simulink model "eVTOL_System"  (R2024b)
settings: Solver=FixedStepAuto  StartTime=0.0  StopTime=inf  RelTol=1e-3
undefined symbols (not defined in the file): airspeed, Battery, BCE12, BCE_Set_init, BMS_Controller_State, C, Cell10_P, Cell11_P, Cell12_P, Cell13_P, Cell14_P, Cell15_P, Cell16_P, Cell17_P, Cell18_P, Cell19_P, Cell1_N, Cell1_P, Cell20_P, Cell21_P, Cell22_P, Cell23_P, Cell24_P, Cell2_P, Cell3_P, Cell4_P, Cell5_P, Cell6_P, Cell7_P, Cell8_P, Cell9_P, Charging_State, CityMission, control, controlParams, ControlSampleTime, CriticalTiltAngle, currentFactor, CV_Gain, ddx, ddy, ddz, Device_01, Device_02, DiscIntNeverNeededParam, dx, dy, dz, Earth, env, F, F28379D_ADC_MaxCount, F28379D_ADC_Vmax, FixedWingMission, flightState, Foc_Ki_IxTcpu, Foc_Ki_S, Foc_Kp_I, Foc_Kp_S, fractalcoef ... (+68)
libraries: fl_lib x1115, nesl_utility x617, slrealtimeethercatlib x217, simulink x130, canmsglib x101, speedgoatlib_IO611_obsolete x91, slpidlib x49, mcbcontrolslib x44, slrealtimeutilitieslib x35, speedgoatlib_hdlCoder_IO3xx x31, dspstat3 x24, mcbpositiondecoderlib x12
(part 9 of 31)

== system eVTOL_System/Battery System/BMS/HIL/Controller_76Cells/Current Calculations ==
  BMS_Input : Inport
  Bus Selector : BusSelector  OutputSignals=Cell_Voltages,Cell_Temperatures
  Charge_Current_Limit_Calc : Subsystem
  Discharge_Current_Limit_Calc : Subsystem
  MinMax : MinMax
  MinMax1 : MinMax
  MinMax2 : MinMax  Function=max
  MinMax4 : MinMax  Function=max
  Selector1 : Subsystem
  Selector3 : Subsystem
  Discharge_Current_Limit : Outport
  Charge_Current_Limit : Outport  Port=2
  wires:
  MinMax/1 -> Discharge_Current_Limit_Calc/1(MinCellVolt)  "Min_Cell_Volt"
  MinMax4/1 -> Discharge_Current_Limit_Calc/3(MaxCellTemp), Charge_Current_Limit_Calc/3(MaxCellTemp)  "Max_Cell_Temp"
  MinMax1/1 -> Discharge_Current_Limit_Calc/2(MinCellTemp), Charge_Current_Limit_Calc/2(MinCellTemp)  "Min_Cell_Temp"
  MinMax2/1 -> Charge_Current_Limit_Calc/1(MaxCellVolt)  "Max_Cell_Volt"
  Discharge_Current_Limit_Calc/1(Discharge_Current_Limit) -> Discharge_Current_Limit/1  "Discharge_Current_Limit"
  Charge_Current_Limit_Calc/1(Charge_Current_Limit) -> Charge_Current_Limit/1  "Charge_Current_Limit"
  Bus Selector/1 -> Selector3/1(In1)  "<Cell_Voltages>"
  Bus Selector/2 -> Selector1/1(In1)  "<Cell_Temperatures>"
  BMS_Input/1 -> Bus Selector/1
  Selector3/1(Out1) -> MinMax/1, MinMax2/1
  Selector1/1(Out1) -> MinMax4/1, MinMax1/1

== system eVTOL_System/Battery System/BMS/HIL/Controller_76Cells/SOC Calculation ==
  BMS_State : Inport  OutDataTypeStr=Enum: BMS_Controller_State
  Sensor_Values : Inport  Port=2
  Bus Selector2 : BusSelector  OutputSignals=Pack_Current,Cell_Voltages,Cell_Temperatures
  Compare To Constant : simulink/Logic and Bit Operations/Compare To Constant  relop=~=  const=BMS_Controller_State.BMS_Fault  OutDataTypeStr=boolean
  Coulomb Counting : Subsystem  VariantControl=SocAlgo==1
  Gain : Gain  Gain=100
  Measurement Function : Subsystem  TreatAsAtomicUnit=on
  Mux : Mux  Inputs=3
  PackCurrent : Gain  Gain=-1
  Selector : Subsystem
  Selector1 : Subsystem
  State Transition Function : Subsystem  TreatAsAtomicUnit=on
  Temp : Selector  InputPortWidth=76  IndexOptions=Index vector (dialog)  Indices=1  OutputSizes=1
  UKF_EKF_1TC : Subsystem  VariantControl=CellType==1
  Volt : Selector  InputPortWidth=76  IndexOptions=Index vector (dialog)  Indices=1  OutputSizes=1
  SOC : Outport  OutDataTypeStr=single  VectorParamsAs1DForOutWhenUnconnected=off
  wires:
  Mux/1 -> Gain/1  "SOC"
  UKF_EKF_1TC/1(SOC_UKF) -> Mux/2  "SOC_UKF"
  BMS_State/1 -> Compare To Constant/1
  Coulomb Counting/1(SOC) -> Mux/1  "SOC_CC"
  Volt/1 -> UKF_EKF_1TC/1(Cell_Voltage)
  Temp/1 -> Coulomb Counting/2(Temp), State Transition Function/2(Temperature K), Measurement Function/2(Temperature (K))
  Compare To Constant/1 -> UKF_EKF_1TC/Enable
  UKF_EKF_1TC/2(SOC_EKF) -> Mux/3  "SOC_EKF"
  Bus Selector2/1 -> Coulomb Counting/1(Curr), PackCurrent/1  "<Pack_Current>"
  PackCurrent/1 -> State Transition Function/1(Current), Measurement Function/1(Current)  "PackCurrent"
  Bus Selector2/3 -> Selector1/1(In1)  "<Cell_Temperatures>"
  Bus Selector2/2 -> Selector/1(In1)  "<Cell_Voltages>"
  Sensor_Values/1 -> Bus Selector2/1
  Gain/1 -> SOC/1
  Selector/1(Out1) -> Volt/1
  Selector1/1(Out1) -> Temp/1

== system eVTOL_System/Battery System/BMS/MIL/Cell Monitoring Unit/Balancing_Circuit ==
  Bal_Cmd_Controller : Inport
  24-Cell : Subsystem  VariantControl=Ns_Module == 12
  Cells : PMIOPort  Side=Left
  Balancing_Currents : Outport
  wires:
  Bal_Cmd_Controller/1 -> 24-Cell/1(Bal_Cmd_Controller)
  24-Cell/1(Balancing_Currents) -> Balancing_Currents/1
  connections:
  Cells/RConn1 -- 24-Cell/LConn1

== system eVTOL_System/Battery System/BMS/MIL/Cell Monitoring Unit/Balancing_Circuit1 ==
  Bal_Cmd_Controller : Inport
  38-Cell : Subsystem  VariantControl=Ns_Module == 12
  Cells : PMIOPort  Side=Left
  Balancing_Currents : Outport
  wires:
  Bal_Cmd_Controller/1 -> 38-Cell/1(Bal_Cmd_Controller)
  38-Cell/1(Balancing_Currents) -> Balancing_Currents/1
  connections:
  Cells/RConn1 -- 38-Cell/LConn1

== system eVTOL_System/Battery System/BMS/MIL/Cell Monitoring Unit/Balancing_Circuit2 ==
  Bal_Cmd_Controller : Inport
  38-Cell : Subsystem  VariantControl=Ns_Module == 12
  Cells : PMIOPort  Side=Left
  Balancing_Currents : Outport
  wires:
  Bal_Cmd_Controller/1 -> 38-Cell/1(Bal_Cmd_Controller)
  38-Cell/1(Balancing_Currents) -> Balancing_Currents/1
  connections:
  Cells/RConn1 -- 38-Cell/LConn1

== system eVTOL_System/Battery System/BMS/MIL/Controller/BMS State Machine ==
  Discharge_Current_Limit : Inport
  Charge_Current_Limit : Inport  Port=2
  State_Request : Inport  Port=3  OutDataTypeStr=Enum: SRE
  Sensor_Values : Inport  Port=4
  Fault_Reset_Enable : Inport  Port=5
  Bus Selector : BusSelector  OutputSignals=Cell_Voltages,Pack_Voltage,Cell_Temperatures,Pack_Current
  Data Type Conversion : DataTypeConversion  OutDataTypeStr=boolean  SaturateOnIntegerOverflow=off  RndMeth=Floor
  State_Machine : Stateflow chart  TreatAsAtomicUnit=on  VariantControl=(default)
  Charge_Current_Req : Outport  OutMin=-100  OutMax=100  OutDataTypeStr=single  VectorParamsAs1DForOutWhenUnconnected=off
  Faults : Outport  Port=2  OutDataTypeStr=Bus: Faults  VectorParamsAs1DForOutWhenUnconnected=off  BusOutputAsStruct=on
  Charging_State : Outport  Port=3
  BMS_State : Outport  Port=4  OutDataTypeStr=Enum: BMS_Controller_State  VectorParamsAs1DForOutWhenUnconnected=off
  wires:
  State_Machine/2(Fault_out) -> Faults/1  "Faults"
  Bus Selector/1 -> State_Machine/4(Cell_Voltages)  "<Cell_Voltages>"
  State_Machine/1(ChargeCurrentReq) -> Charge_Current_Req/1  "Charge_Current_Req"
  State_Request/1 -> State_Machine/3(State_Request)
  Discharge_Current_Limit/1 -> State_Machine/1(DischargeCurrentLimit)
  Charge_Current_Limit/1 -> State_Machine/2(ChargeCurrentLimit)
  Bus Selector/3 -> State_Machine/6(Cell_Temperatures)  "<Cell_Temperatures>"
  Bus Selector/2 -> State_Machine/5(Pack_Voltage)  "<Pack_Voltage>"
  Bus Selector/4 -> State_Machine/7(Pack_Current)  "<Pack_Current>"
  Sensor_Values/1 -> Bus Selector/1
  Fault_Reset_Enable/1 -> Data Type Conversion/1
  Data Type Conversion/1 -> State_Machine/8(Fault_Reset_Enable)
  State_Machine/3(ChargeModeReq) -> Charging_State/1  "Charging_State"
  State_Machine/4(BMS_State) -> BMS_State/1  "BMS_State"

== system eVTOL_System/Battery System/BMS/MIL/Controller/Balancing Logic ==
  BMS_State : Inport  OutDataTypeStr=Enum: BMS_Controller_State  PortDimensions=1
  Sensor_Values : Inport  Port=2
  Balancing : Stateflow chart  TreatAsAtomicUnit=on  VariantControl=(default)
  Bus Selector1 : BusSelector  OutputSignals=Cell_Voltages
  Bal_Cmd : Outport  OutDataTypeStr=boolean  PortDimensions=[1,NumModules*Ns_Module]  VectorParamsAs1DForOutWhenUnconnected=off
  wires:
  Balancing/1(Bal_Cmd) -> Bal_Cmd/1  "Bal_Cmd"
  Bus Selector1/1 -> Balancing/2(CellVoltages)  "<Cell_Voltages>"
  Sensor_Values/1 -> Bus Selector1/1
  BMS_State/1 -> Balancing/1(BMS_State)

== system eVTOL_System/Battery System/BMS/MIL/Controller/Current Calculations ==
  BMS_Input : Inport
  Bus Selector : BusSelector  OutputSignals=Cell_Voltages,Cell_Temperatures
  Charge_Current_Limit_Calc : Subsystem
  Discharge_Current_Limit_Calc : Subsystem
  MinMax : MinMax
  MinMax1 : MinMax
  MinMax2 : MinMax  Function=max
  MinMax4 : MinMax  Function=max
  Discharge_Current_Limit : Outport
  Charge_Current_Limit : Outport  Port=2
  wires:
  MinMax/1 -> Discharge_Current_Limit_Calc/1(MinCellVolt)  "Min_Cell_Volt"
  MinMax4/1 -> Discharge_Current_Limit_Calc/3(MaxCellTemp), Charge_Current_Limit_Calc/3(MaxCellTemp)  "Max_Cell_Temp"
  MinMax1/1 -> Discharge_Current_Limit_Calc/2(MinCellTemp), Charge_Current_Limit_Calc/2(MinCellTemp)  "Min_Cell_Temp"
  MinMax2/1 -> Charge_Current_Limit_Calc/1(MaxCellVolt)  "Max_Cell_Volt"
  Discharge_Current_Limit_Calc/1(Discharge_Current_Limit) -> Discharge_Current_Limit/1  "Discharge_Current_Limit"
  Charge_Current_Limit_Calc/1(Charge_Current_Limit) -> Charge_Current_Limit/1  "Charge_Current_Limit"
  Bus Selector/1 -> MinMax/1, MinMax2/1  "<Cell_Voltages>"
  Bus Selector/2 -> MinMax4/1, MinMax1/1  "<Cell_Temperatures>"
  BMS_Input/1 -> Bus Selector/1

== system eVTOL_System/Battery System/BMS/MIL/Controller/SOC Calculation ==
  BMS_State : Inport  OutDataTypeStr=Enum: BMS_Controller_State
  Sensor_Values : Inport  Port=2
  Bus Selector2 : BusSelector  OutputSignals=Pack_Current,Cell_Voltages,Cell_Temperatures
  Compare To Constant : simulink/Logic and Bit Operations/Compare To Constant  relop=~=  const=BMS_Controller_State.BMS_Fault  OutDataTypeStr=boolean
  Coulomb Counting : Subsystem  VariantControl=SocAlgo==1
  Gain : Gain  Gain=100
  Measurement Function : Subsystem  TreatAsAtomicUnit=on
  Mux : Mux  Inputs=3
  PackCurrent : Gain  Gain=-1
  State Transition Function : Subsystem  TreatAsAtomicUnit=on
  Temp : Selector  InputPortWidth=Ns_Module*NumModules  IndexOptions=Index vector (dialog)  Indices=1  OutputSizes=1
  UKF_EKF_1TC : Subsystem  VariantControl=CellType==1
  Volt : Selector  InputPortWidth=Ns_Module*NumModules  IndexOptions=Index vector (dialog)  Indices=1  OutputSizes=1
  SOC : Outport  OutDataTypeStr=single  VectorParamsAs1DForOutWhenUnconnected=off
  wires:
  Mux/1 -> Gain/1  "SOC"
  UKF_EKF_1TC/1(SOC_UKF) -> Mux/2  "SOC_UKF"
  BMS_State/1 -> Compare To Constant/1
  Coulomb Counting/1(SOC) -> Mux/1  "SOC_CC"
  Volt/1 -> UKF_EKF_1TC/1(Cell_Voltage)
  Temp/1 -> Coulomb Counting/2(Temp), State Transition Function/2(Temperature K), Measurement Function/2(Temperature (K))
  Compare To Constant/1 -> UKF_EKF_1TC/Enable
  UKF_EKF_1TC/2(SOC_EKF) -> Mux/3  "SOC_EKF"
  Bus Selector2/1 -> Coulomb Counting/1(Curr), PackCurrent/1  "<Pack_Current>"
  PackCurrent/1 -> State Transition Function/1(Current), Measurement Function/1(Current)  "PackCurrent"
  Bus Selector2/3 -> Temp/1  "<Cell_Temperatures>"
  Bus Selector2/2 -> Volt/1  "<Cell_Voltages>"
  Sensor_Values/1 -> Bus Selector2/1
  Gain/1 -> SOC/1

== system eVTOL_System/Battery System/Battery/Battery Pack/100-Cell/Faults ==
  note: Short-Circuits
  note: Short-Circuits
  Short_Circuits : Inport
  Array of Electrical Nodes Connector : batt_lib/Connectors/Array of Electrical Nodes Connector  numInputConnections=simscape.battery.enum.thermal.numArrayOfNodesConnections.twentyfour  inNode1NumElements=1  inNode2NumElements=1  inNode3NumElements=1  inNode4NumElements=1  inNode5NumElements=1  inNode6NumElements=1  inNode7NumElements=1  inNode8NumElements=1  inNode9NumElements=1  inNode10NumElements=1  inNode11NumElements=1  inNode12NumElements=1  inNode13NumElements=1  inNode14NumElements=1  inNode15NumElements=1  inNode16NumElements=1  inNode17NumElements=1  inNode18NumElements=1  inNode19NumElements=1  inNode20NumElements=1  inNode21NumElements=1  inNode22NumElements=1  inNode23NumElements=1  inNode24NumElements=1  inNode25NumElements=1  inNode26NumElements=1  inNode27NumElements=1  inNode28NumElements=1  inNode29NumElements=1  inNode30NumElements=1  inNode31NumElements=1  inNode32NumElements=1  inNode33NumElements=1  inNode34NumElements=1  inNode35NumElements=1  inNode36NumElements=1  inNode37NumElements=1  inNode38NumElements=1  inNode39NumElements=1  inNode40NumElements=1  inNode41NumElements=1  inNode42NumElements=1  inNode43NumElements=1  inNode44NumElements=1  inNode45NumElements=1  inNode46NumElements=1  inNode47NumElements=1  inNode48NumElements=1  inNode49NumElements=1  inNode50NumElements=1
      settings: InternalSimscapePortConfiguration="{\"Bottom\":[{\"id\":\"outConn\",\"label\":\"outConn\",\"type\":\"foundation.electrical.electrical\"}],\"Left\":[],\"Right\":[],\"Top\":[{\"id\":\"inConn1\",\"label\":\"inConn1\",\"type\":\"foundation.electrical.electrical\"},{\"id\":\"inConn2\",\"label\":\"inConn2\",\"type\":\"foundation.electrical.electrical\"},{\"id\":\"inConn3\",\"label\":\"inConn3\",\"type\":\"foundation.electrical.electrical\"},{\"id\":\"inConn4\",\"label\":\"inConn4\",\"type\":\"foundation.electrical.electrical\"},{\"id\":\"inConn5\",\"label\":\"inConn5\",\"type\":\"foundation.electrical.electrical\"},{\"id\":\"inConn6\",\"label\":\"inConn6\",\"type\":\"foundation.electrical.electrical\"},{\"id\":\"inConn7\",\"label\":\"inConn7\",\"type\":\"foundation.electrical.electrical\"},{\"id\":\"inConn8\",\"label\":\"inConn8\",\"type\":\"foundation.electrical.electrical\"},{\"id\":\"inConn9\",\"label\":\"inConn9\",\"type\":\"foundation.electrical.electrical\"},{\"id\":\"inConn10\",\"label\":\"inConn10\",\"type\":\"foundation.electrical.electrical\"},{\"id\":\"inConn11\",\"label\":\"inConn11\",\"type\":\"foundation.electrical.electrical\"},{\"id\":\"inConn12\",\"label\":\"inConn12\",\"type\":\"foundation.electrical.electrical\"},{\"id\":\"inConn13\",\"label\":\"inConn13\",\"type\":\"foundation.electrical.electrical\"},{\"id\":\"inConn14\",\"label\":\"inConn14\",\"type\":\"foundation.electrical.electrical\"},{\"id\":\"inConn15\",\"label\":\"inConn15\",\"type\":\"foundation.electrical.electrical\"},{\"id\":\"inConn16\",\"label\":\"inConn16\",\"type\":\"foundation.electrical.electrical\"},{\"id\":\"inConn17\",\"label\":\"inConn17\",\"type\":\"foundation.electrical.electrical\"},{\"id\":\"inConn18\",\"label\":\"inConn18\",\"type\":\"foundation.electrical.electrical\"},{\"id\":\"inConn19\",\"label\":\"inConn19\",\"type\":\"foundation.electrical.electrical\"},{\"id\":\"inConn20\",\"label\":\"inConn20\",\"type\":\"foundation.electrical.electrical\"},{\"id\":\"inConn21\",\"label\":\"inConn21\",\"type\":\"foundation.electrical.electrical\"},{\"id\":\"inConn22\",\"label\":\"inConn22\",\"type\":\"foundation.electrical.electrical\"},{\"id\":\"inConn23\",\"label\":\"inConn23\",\"type\":\"foundation.electrical.electrical\"},{\"id\":\"inConn24\",\"label\":\"inConn24\",\"type\":\"foundation.electrical.electrical\"}]}"
  Connection Label : ConnectionLabel  Label=pos1
  Connection Label1 : ConnectionLabel  Label=pos7
  Connection Label10 : ConnectionLabel  Label=pos3
  Connection Label11 : ConnectionLabel  Label=pos2
  Connection Label12 : ConnectionLabel  Label=pos12
  Connection Label13 : ConnectionLabel  Label=pos11
  Connection Label14 : ConnectionLabel  Label=pos10
  Connection Label15 : ConnectionLabel  Label=pos9
  Connection Label16 : ConnectionLabel  Label=pos8
  Connection Label17 : ConnectionLabel  Label=pos7
  Connection Label18 : ConnectionLabel  Label=pos6
  Connection Label19 : ConnectionLabel  Label=pos5
  Connection Label2 : ConnectionLabel  Label=pos8
  Connection Label20 : ConnectionLabel  Label=pos4
  Connection Label21 : ConnectionLabel  Label=pos3
  Connection Label22 : ConnectionLabel  Label=pos2
  Connection Label23 : ConnectionLabel  Label=pos1
  Connection Label3 : ConnectionLabel  Label=pos9
  Connection Label4 : ConnectionLabel  Label=pos10
  Connection Label48 : ConnectionLabel  Label=pos24
  Connection Label49 : ConnectionLabel  Label=pos23
  Connection Label5 : ConnectionLabel  Label=pos11
  Connection Label50 : ConnectionLabel  Label=pos22
  Connection Label51 : ConnectionLabel  Label=pos21
  Connection Label52 : ConnectionLabel  Label=pos20
  Connection Label53 : ConnectionLabel  Label=pos19
  Connection Label54 : ConnectionLabel  Label=pos18
  Connection Label55 : ConnectionLabel  Label=pos17
  Connection Label56 : ConnectionLabel  Label=pos16
  Connection Label57 : ConnectionLabel  Label=pos15
  Connection Label58 : ConnectionLabel  Label=pos14
  Connection Label59 : ConnectionLabel  Label=pos13
  Connection Label6 : ConnectionLabel  Label=pos12
  Connection Label60 : ConnectionLabel  Label=pos13
  Connection Label61 : ConnectionLabel  Label=pos19
  Connection Label62 : ConnectionLabel  Label=pos15
  Connection Label63 : ConnectionLabel  Label=pos14
  Connection Label64 : ConnectionLabel  Label=pos20
  Connection Label65 : ConnectionLabel  Label=pos21
  Connection Label66 : ConnectionLabel  Label=pos22
  Connection Label67 : ConnectionLabel  Label=pos23
  Connection Label68 : ConnectionLabel  Label=pos24
  Connection Label69 : ConnectionLabel  Label=pos18
  Connection Label7 : ConnectionLabel  Label=pos6
  Connection Label70 : ConnectionLabel  Label=pos17
  Connection Label71 : ConnectionLabel  Label=pos16
  Connection Label8 : ConnectionLabel  Label=pos5
  Connection Label9 : ConnectionLabel  Label=pos4
  Data Type Conversion1 : DataTypeConversion  OutDataTypeStr=double  SaturateOnIntegerOverflow=off  RndMeth=Floor
  Selector1 : Selector  IndexOptions=Index vector (dialog)  Indices=2  OutputSizes=1
  Selector10 : Selector  IndexOptions=Index vector (dialog)  Indices=12  OutputSizes=1
  Selector11 : Selector  IndexOptions=Index vector (dialog)  Indices=11  OutputSizes=1
  Selector12 : Selector  IndexOptions=Index vector (dialog)  Indices=9  OutputSizes=1
  Selector13 : Selector  IndexOptions=Index vector (dialog)  Indices=14  OutputSizes=1
  Selector14 : Selector  IndexOptions=Index vector (dialog)  Indices=24  OutputSizes=1
  Selector15 : Selector  IndexOptions=Index vector (dialog)  Indices=23  OutputSizes=1
  Selector16 : Selector  IndexOptions=Index vector (dialog)  Indices=21  OutputSizes=1
  Selector17 : Selector  IndexOptions=Index vector (dialog)  Indices=16  OutputSizes=1
  Selector18 : Selector  IndexOptions=Index vector (dialog)  Indices=15  OutputSizes=1
  Selector19 : Selector  IndexOptions=Index vector (dialog)  Indices=18  OutputSizes=1
  Selector2 : Selector  IndexOptions=Index vector (dialog)  Indices=4  OutputSizes=1
  Selector20 : Selector  IndexOptions=Index vector (dialog)  Indices=20  OutputSizes=1
  Selector21 : Selector  IndexOptions=Index vector (dialog)  Indices=13  OutputSizes=1
  Selector22 : Selector  IndexOptions=Index vector (dialog)  Indices=19  OutputSizes=1
  Selector23 : Selector  IndexOptions=Index vector (dialog)  Indices=17  OutputSizes=1
  Selector24 : Selector  IndexOptions=Index vector (dialog)  Indices=22  OutputSizes=1
  Selector3 : Selector  IndexOptions=Index vector (dialog)  Indices=3  OutputSizes=1
  Selector4 : Selector  IndexOptions=Index vector (dialog)  Indices=6  OutputSizes=1
  Selector5 : Selector  IndexOptions=Index vector (dialog)  Indices=8  OutputSizes=1
  Selector6 : Selector  IndexOptions=Index vector (dialog)  Indices=1  OutputSizes=1
  Selector7 : Selector  IndexOptions=Index vector (dialog)  Indices=7  OutputSizes=1
  Selector8 : Selector  IndexOptions=Index vector (dialog)  Indices=5  OutputSizes=1
  Selector9 : Selector  IndexOptions=Index vector (dialog)  Indices=10  OutputSizes=1
  Simscape Bus : SimscapeBus  HierarchyStrings=Cell24_P;Cell23_P;Cell22_P;Cell21_P;Cell20_P;Cell19_P;Cell18_P;Cell17_P;Cell16_P;Cell15_P;Cell14_P;Cell13_P;Cell12_P;Cell11_P;Cell10_P;Cell9_P;Cell8_P;Cell7_P;Cell6_P;Cell5_P;Cell4_P;Cell3_P;Cell2_P;Cell1_P;Cell1_N
  Simulink-PS Converter{1..12,14..25} (24 alike) : nesl_utility/Simulink-PS Converter  PhysicalDomain=network_engine_domain  SubClassName=ps_input  LeftPortType=input  RightPortType=output  PseudoPeriodic=off  Frequencies=[]  NoiseDistribution=none  NoiseParameters=[]  Unit=1  AffineConversion=off  FilteringAndDerivatives=zero  SimscapeFilterOrder=1  InputFilterTimeConstant=0.001  UdotUserProvided=1
  Switch{,1..23} (24 alike) : fl_lib/Electrical/Electrical Elements/Switch  R_closed=0.01 Ohm  G_open=1e-8 1/Ohm  Threshold=0.5  i_specify=off  i_priority=None  i=0 A  i_nominal_specify=off  i_nominal_value=1  i_nominal_unit=A  v_specify=off  v_priority=None  v=0 V  v_nominal_specify=off  v_nominal_value=1  v_nominal_unit=V
  +Bus : PMIOPort  Side=Right
  Cells : PMIOPort  Port=2  Side=Right
  =Bus : PMIOPort  Port=3  Side=Right
  wires:
  [Cell13_Switch_SC] -> Simulink-PS Converter14/1
  [Cell14_Switch_SC] -> Simulink-PS Converter15/1
  [Cell21_Switch_SC] -> Simulink-PS Converter22/1
  [Cell17_Switch_SC] -> Simulink-PS Converter18/1
  [Cell20_Switch_SC] -> Simulink-PS Converter21/1
  [Cell15_Switch_SC] -> Simulink-PS Converter16/1
  [Cell16_Switch_SC] -> Simulink-PS Converter17/1
  [Cell19_Switch_SC] -> Simulink-PS Converter20/1
  [Cell18_Switch_SC] -> Simulink-PS Converter19/1
  Short_Circuits/1 -> Data Type Conversion1/1
  [Cell9_Switch_SC] -> Simulink-PS Converter9/1
  [Cell6_Switch_SC] -> Simulink-PS Converter6/1
  [Cell3_Switch_SC] -> Simulink-PS Converter3/1
  [Cell4_Switch_SC] -> Simulink-PS Converter4/1
  [Cell12_Switch_SC] -> Simulink-PS Converter12/1
  [Cell5_Switch_SC] -> Simulink-PS Converter5/1
  [Cell11_Switch_SC] -> Simulink-PS Converter11/1
  [Cell8_Switch_SC] -> Simulink-PS Converter8/1
  [Cell1_Switch_SC] -> Simulink-PS Converter1/1
  [Cell10_Switch_SC] -> Simulink-PS Converter10/1
  [Cell7_Switch_SC] -> Simulink-PS Converter7/1
  [Cell2_Switch_SC] -> Simulink-PS Converter2/1
  Data Type Conversion1/1 -> Selector4/1, Selector2/1, Selector3/1, Selector6/1, Selector1/1, Selector8/1, Selector7/1, Selector5/1, Selector12/1, Selector9/1, Selector11/1, Selector16/1, Selector24/1, Selector15/1, Selector14/1, Selector20/1, Selector22/1, Selector19/1, Selector23/1, Selector17/1, Selector18/1, Selector13/1, Selector21/1, Selector10/1
  Selector6/1 -> [Cell1_Switch_SC]
  Selector1/1 -> [Cell2_Switch_SC]
  Selector3/1 -> [Cell3_Switch_SC]
  Selector2/1 -> [Cell4_Switch_SC]
  Selector8/1 -> [Cell5_Switch_SC]
  Selector4/1 -> [Cell6_Switch_SC]
  Selector7/1 -> [Cell7_Switch_SC]
  Selector5/1 -> [Cell8_Switch_SC]
  Selector12/1 -> [Cell9_Switch_SC]
  Selector9/1 -> [Cell10_Switch_SC]
  Selector11/1 -> [Cell11_Switch_SC]
  Selector10/1 -> [Cell12_Switch_SC]
  Selector21/1 -> [Cell13_Switch_SC]
  Selector13/1 -> [Cell14_Switch_SC]
  Selector18/1 -> [Cell15_Switch_SC]
  Selector17/1 -> [Cell16_Switch_SC]
  Selector23/1 -> [Cell17_Switch_SC]
  Selector19/1 -> [Cell18_Switch_SC]
  Selector22/1 -> [Cell19_Switch_SC]
  Selector20/1 -> [Cell20_Switch_SC]
  Selector16/1 -> [Cell21_Switch_SC]
  Selector24/1 -> [Cell22_Switch_SC]
  Selector15/1 -> [Cell23_Switch_SC]
  Selector14/1 -> [Cell24_Switch_SC]
  [Cell24_Switch_SC] -> Simulink-PS Converter25/1
  [Cell23_Switch_SC] -> Simulink-PS Converter24/1
  [Cell22_Switch_SC] -> Simulink-PS Converter23/1
  connections:
  Simulink-PS Converter17/RConn1 -- Switch3/RConn1
  Switch3/LConn1 -- Connection Label56/LConn1 -- Switch2/RConn2 -- Simscape Bus/LConn16
  Switch6/LConn1 -- Simscape Bus/LConn19 -- Connection Label53/LConn1 -- Switch5/RConn2
  Switch7/LConn1 -- Simscape Bus/LConn20 -- Connection Label52/LConn1 -- Switch6/RConn2
  Switch2/LConn1 -- Connection Label57/LConn1 -- Switch1/RConn2 -- Simscape Bus/LConn15
  Simulink-PS Converter16/RConn1 -- Switch2/RConn1
  Simulink-PS Converter19/RConn1 -- Switch5/RConn1
  Switch10/LConn1 -- Simscape Bus/LConn23 -- Connection Label49/LConn1 -- Switch9/RConn2
  Simulink-PS Converter25/RConn1 -- Switch11/RConn1
  Switch11/LConn1 -- Simscape Bus/LConn24 -- Connection Label48/LConn1 -- Switch10/RConn2
  Switch9/LConn1 -- Simscape Bus/LConn22 -- Connection Label50/LConn1 -- Switch8/RConn2
  Simulink-PS Converter14/RConn1 -- Switch/RConn1
  Simscape Bus/LConn25 -- Switch11/RConn2
  Simulink-PS Converter18/RConn1 -- Switch4/RConn1
  Switch4/LConn1 -- Connection Label55/LConn1 -- Switch3/RConn2 -- Simscape Bus/LConn17
  Simulink-PS Converter24/RConn1 -- Switch10/RConn1
  Switch8/LConn1 -- Simscape Bus/LConn21 -- Connection Label51/LConn1 -- Switch7/RConn2
  Simulink-PS Converter20/RConn1 -- Switch6/RConn1
  Simulink-PS Converter15/RConn1 -- Switch1/RConn1
  Simulink-PS Converter21/RConn1 -- Switch7/RConn1
  Simulink-PS Converter23/RConn1 -- Switch9/RConn1
  Simulink-PS Converter22/RConn1 -- Switch8/RConn1
  Switch5/LConn1 -- Simscape Bus/LConn18 -- Connection Label54/LConn1 -- Switch4/RConn2
  Switch15/RConn2 -- Simscape Bus/LConn13 -- Switch/LConn1 -- Connection Label59/LConn1
  Switch1/LConn1 -- Simscape Bus/LConn14 -- Connection Label58/LConn1 -- Switch/RConn2
  Array of Electrical Nodes Connector/RConn1 -- +Bus/RConn1
  Switch17/LConn1 -- Simscape Bus/LConn4 -- Connection Label20/LConn1 -- Switch16/RConn2
  Switch14/LConn1 -- Simscape Bus/LConn11 -- Connection Label13/LConn1 -- Switch23/RConn2
  Simscape Bus/LConn6 -- Switch19/LConn1 -- Connection Label18/LConn1 -- Switch18/RConn2
  Switch13/LConn1 -- Simscape Bus/LConn2 -- Connection Label22/LConn1 -- Switch12/RConn2
  Switch22/LConn1 -- Simscape Bus/LConn9 -- Connection Label15/LConn1 -- Switch21/RConn2
  Switch18/LConn1 -- Simscape Bus/LConn5 -- Connection Label19/LConn1 -- Switch17/RConn2
  Switch13/RConn2 -- Connection Label21/LConn1 -- Switch16/LConn1 -- Simscape Bus/LConn3
  Simscape Bus/LConn1 -- Connection Label23/LConn1 -- Switch12/LConn1
  Switch21/LConn1 -- Simscape Bus/LConn8 -- Connection Label16/LConn1 -- Switch20/RConn2
  Switch20/LConn1 -- Simscape Bus/LConn7 -- Connection Label17/LConn1 -- Switch19/RConn2
  Simulink-PS Converter12/RConn1 -- Switch15/RConn1
  Simulink-PS Converter7/RConn1 -- Switch20/RConn1
  Simulink-PS Converter10/RConn1 -- Switch23/RConn1
  Simulink-PS Converter2/RConn1 -- Switch13/RConn1
  Simulink-PS Converter3/RConn1 -- Switch16/RConn1
  Simulink-PS Converter1/RConn1 -- Switch12/RConn1
  Simulink-PS Converter11/RConn1 -- Switch14/RConn1
  Simulink-PS Converter8/RConn1 -- Switch21/RConn1
  Simulink-PS Converter9/RConn1 -- Switch22/RConn1
  Simulink-PS Converter5/RConn1 -- Switch18/RConn1
  Simulink-PS Converter6/RConn1 -- Switch19/RConn1
  Simulink-PS Converter4/RConn1 -- Switch17/RConn1
  Switch15/LConn1 -- Simscape Bus/LConn12 -- Switch14/RConn2 -- Connection Label12/LConn1
  Simscape Bus/LConn10 -- Connection Label14/LConn1 -- Switch22/RConn2 -- Switch23/LConn1
  Cells/RConn1 -- Simscape Bus/RConn1
  Connection Label/LConn1 -- Array of Electrical Nodes Connector/LConn1
  Connection Label11/LConn1 -- Array of Electrical Nodes Connector/LConn2
  Connection Label10/LConn1 -- Array of Electrical Nodes Connector/LConn3
  Connection Label9/LConn1 -- Array of Electrical Nodes Connector/LConn4
  Connection Label8/LConn1 -- Array of Electrical Nodes Connector/LConn5
  Connection Label7/LConn1 -- Array of Electrical Nodes Connector/LConn6
  Connection Label1/LConn1 -- Array of Electrical Nodes Connector/LConn7
  Connection Label2/LConn1 -- Array of Electrical Nodes Connector/LConn8
  Connection Label3/LConn1 -- Array of Electrical Nodes Connector/LConn9
  Connection Label4/LConn1 -- Array of Electrical Nodes Connector/LConn10
  Connection Label5/LConn1 -- Array of Electrical Nodes Connector/LConn11
  Connection Label6/LConn1 -- Array of Electrical Nodes Connector/LConn12
  Connection Label60/LConn1 -- Array of Electrical Nodes Connector/LConn13
  Connection Label63/LConn1 -- Array of Electrical Nodes Connector/LConn14
  Connection Label62/LConn1 -- Array of Electrical Nodes Connector/LConn15
  Connection Label71/LConn1 -- Array of Electrical Nodes Connector/LConn16
  Connection Label70/LConn1 -- Array of Electrical Nodes Connector/LConn17
  Connection Label69/LConn1 -- Array of Electrical Nodes Connector/LConn18
  Connection Label61/LConn1 -- Array of Electrical Nodes Connector/LConn19
  Connection Label64/LConn1 -- Array of Electrical Nodes Connector/LConn20
  Connection Label65/LConn1 -- Array of Electrical Nodes Connector/LConn21
  Connection Label66/LConn1 -- Array of Electrical Nodes Connector/LConn22
  Connection Label67/LConn1 -- Array of Electrical Nodes Connector/LConn23
  Connection Label68/LConn1 -- Array of Electrical Nodes Connector/LConn24
